simulink model "FuzzyHYPFWMLI"  (R2025a)
settings: Solver=ode23t  StartTime=0.0  StopTime=1  FixedStep=1.0000000100000003E-5  MaxStep=1e-3  RelTol=1e-2  EnableMultiTasking=on
undefined symbols (not defined in the file): c1, c2, c3, c4, c5, c6, DiscIntNeverNeededParam, FC1, FC2, idq1, idq2, PV10k1, PV10k2, PV10k3, R, WM1
libraries: powerlib x93, powerlib_meascontrol x9, fuzblock x8, powerlib_extras x6, re_lib x3, electricdrivelib x2, slpidlib x1
(part 2 of 3)

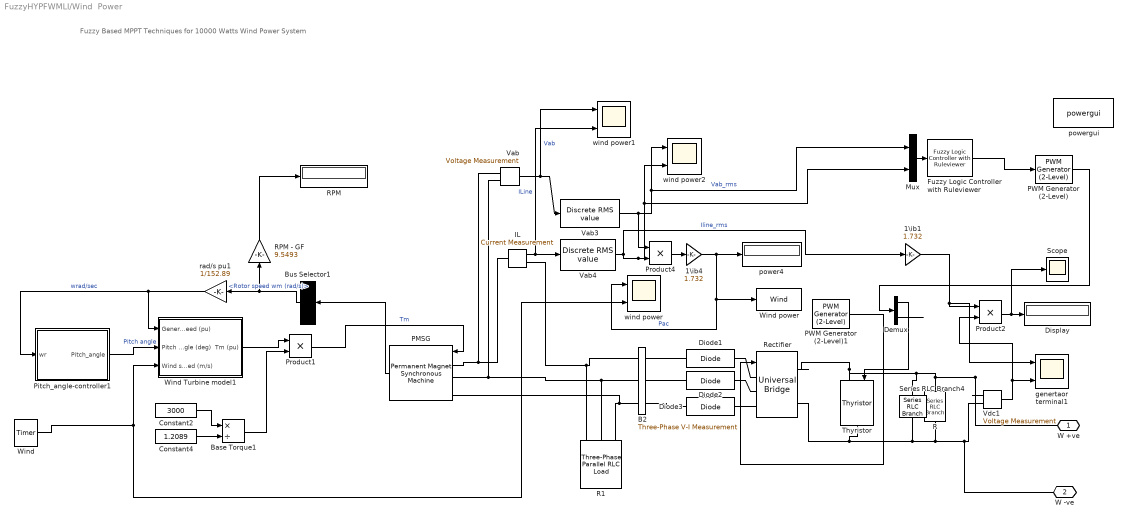
== system FuzzyHYPFWMLI/Wind  Power  ==
  note: Fuzzy Based MPPT Techniques for 10000 Watts Wind Power System
  1\ib1 : Gain  Gain=1.732  SaturateOnIntegerOverflow=on  OutDataTypeStr=Inherit: Same as input  ParamDataTypeStr=Inherit: Same as input
  1\ib4 : Gain  Gain=1.732  SaturateOnIntegerOverflow=on  OutDataTypeStr=Inherit: Same as input  ParamDataTypeStr=Inherit: Same as input
  "B2 " : powerlib/Measurements/Three-Phase V-I Measurement  VoltageMeasurement=no  SetLabelV=on  LabelV=Vabc_B2  Vpu=off  VpuLL=off  CurrentMeasurement=no  SetLabelI=on  LabelI=Iabc_B2  Ipu=off  Pbase=100e6  Vbase=500e3  OutputType=Magnitude  PhasorSimulation=off  PSBequivalent=0
  Base Torque1 : Product  Inputs=*/  RndMeth=Zero
  Bus Selector1 : BusSelector  OutputSignals=Rotor speed wm (rad/s)
  Constant2 : Constant  Value=3000
  Constant4 : Constant  Value=1.2089
  Demux : Demux  Outputs=2
  Diode1 : powerlib/Power Electronics/Diode  Ron=0.001  Lon=0  Vf=0.8  IC=0  UseSnubber=off  Rs=500  Cs=250e-9  Measurements=off
  Diode2 : powerlib/Power Electronics/Diode  Ron=0.001  Lon=0  Vf=0.8  IC=0  UseSnubber=off  Rs=500  Cs=250e-9  Measurements=off
  Diode3 : powerlib/Power Electronics/Diode  Ron=0.001  Lon=0  Vf=0.8  IC=0  UseSnubber=off  Rs=500  Cs=250e-9  Measurements=off
  Display : Display
  Fuzzy Logic Controller with Ruleviewer : fuzblock/Fuzzy Logic  Controller  with Ruleviewer  fismatrix=[WM1]  Ts=0.01
  IL : powerlib/Measurements/Current Measurement  PhasorSimulation=off  OutputType=Complex  PSBequivalent=0
  Mux : Mux  Inputs=2
  PMSG : powerlib/Machines/Permanent Magnet Synchronous Machine  NbPhases=3  FluxDistribution=Sinusoidal  RotorType=Round  MechanicalLoad=Torque Tm  PresetModel=No  ShowDetailedParameters=on  MeasurementBus=off  Resistance=0.0918  Inductance=8.5e-3  dqInductances=[0.0082 0.0082]  La=0.000975  MachineConstant=Flux linkage established by magnets (V.s)  Flux=0.1688  VoltageCst=122.4677  TorqueCst=1.0128  Flat=120  Mechanical=[0.003945 0.0004924 4 0]  PolePairs=4  InitialConditions=[0,0, 0,0]  InitialConditions5ph=[0 0 0 0 0 0]  TsPowergui=0  TsBlock=-1  RefAngle=90 degrees behind phase A axis (modified Park)
      settings: SourceProductName=Simscape Power Systems
  PWM Generator (2-Level) : powerlib_meascontrol/Pulse & Signal Generators/PWM Generator (2-Level)  ModulatorType=Single-phase half-bridge (2 pulses)  ModulatorMode=Unsynchronized  Fc=3000  Pc=90  nF=27  MinMax="[ -1  1 ]"  SamplingTechnique=Natural  ModulatingSignals=off  m=0.8  Freq=60  Phase=0  Ts=0  ShowCarrierOutport=off
      settings: SourceProductName=Simscape Power Systems
  PWM Generator (2-Level)1 : powerlib_meascontrol/Pulse & Signal Generators/PWM Generator (2-Level)  ModulatorType=Three-phase bridge (6 pulses)  ModulatorMode=Unsynchronized  Fc=27*60  Pc=90  nF=27  MinMax="[ -1  1 ]"  SamplingTechnique=Natural  ModulatingSignals=on  m=0.7  Freq=50  Phase=0  Ts=0  ShowCarrierOutport=off
      settings: SourceProductName=Simscape Power Systems
  Pitch_angle-controller1 : Subsystem
  Product1 : Product  RndMeth=Zero
  Product2 : Product  RndMeth=Zero
  Product4 : Product  RndMeth=Zero
  R : powerlib/Elements/Series RLC Branch  LConnTagsString=__new0  RConnTagsString=__new0  BranchType=R  Resistance=10e3  Inductance=1e-3  SetiL0=off  InitialCurrent=0  Capacitance=1e-6  Setx0=off  InitialVoltage=0  Measurements=None
  "R1 " : powerlib/Elements/Three-Phase Parallel RLC Load  LConnTagsString=A|B|C  Configuration=Y (grounded)  NominalVoltage=220  Vabc=[1e3 1e3 1e3]  Vabcp=[1e3 1e3 1e3]  NominalFrequency=50  UnbalancedPower=off  ActivePower=12000  InductivePower=0  CapacitivePower=0  Pabc=[9e3 9e3 9e3]  QLabc=[100 90 110]  QCabc=[100 90 110]  Pabcp=[10e3 9e3 11e3]  QLabcp=[100 90 110]  QCabcp=[100 90 110]  Measurements=None  LoadType=constant Z
  "RPM " : Display
  RPM - GF : Gain  Gain=9.5493  SaturateOnIntegerOverflow=on  OutDataTypeStr=Inherit: Same as input  ParamDataTypeStr=Inherit: Same as input
  Rectifier : powerlib/Power Electronics/Universal Bridge  Arms=3  SnubberResistance=100  SnubberCapacitance=0.1e-6  Device=IGBT / Diodes  Ron=1e-3  Lon=0  ForwardVoltages="[  100  100  ]"  ForwardVoltage=.8  GTOparameters=[ 10e-6 , 20e-6 ]  IGBTparameters=[ 1e-6 , 2e-6 ]  Measurements=Device currents  Measurements_2=None  converterType=Rectifier
  Scope : Scope
      settings: Title=Fuzzy Wind MPPT  ActiveDisplayYMinimum=-1251.33886  ActiveDisplayYMaximum=11262.04974  YLabel=Power ( W )
  Series RLC Branch4 : powerlib/Elements/Series RLC Branch  LConnTagsString=__new0  RConnTagsString=__new0  BranchType=C  Resistance=R  Inductance=1e-3  SetiL0=off  InitialCurrent=0  Capacitance=470e-5  Setx0=off  InitialVoltage=0  Measurements=Branch voltage and current
  Thyristor : powerlib/Power Electronics/Thyristor  Ron=0.001  Lon=0  Vf=220  IC=0  Rs=500  Cs=250e-9  Measurements=off
  Vab : powerlib/Measurements/Voltage Measurement  PhasorSimulation=off  OutputType=Complex  PSBequivalent=0
  Vab3 : powerlib_extras/Discrete Measurements/Discrete  RMS value  Freq=50  Mag_Init=0  Ts=20e-6
  Vab4 : powerlib_extras/Discrete Measurements/Discrete  RMS value  Freq=50  Mag_Init=0  Ts=20e-6
  Vdc1 : powerlib/Measurements/Voltage Measurement  Tag=PoWeRsYsTeMmEaSuReMeNt  PhasorSimulation=off  OutputType=Magnitude  PSBequivalent=0
  "Wind " : powerlib_extras/Control  Blocks/Timer  t=[0 0.05 0.1 0.15 0.2 ]  e=[5 7 11 12 12]
  Wind Turbine model1 : Subsystem  AncestorBlock=DRlib/Wind Generation/Wind Turbine  DialogController=POWERSYS.PowerSysDialog  mask(Wind Turbine){Pnom=10000, Pelec_base=10000/0.9, wind_base=12, P_wind_base=0.8, speed_nom=1, pitch_angle=0, DisplayTurbChar=off, c1_c6=[0.51763          116          0.4            5           21     0.006795], cp_nom=0.48, lambda_nom=8.1}
      mask prompts: Pnom "Nominal mechanical output power (W):"; Pelec_base "Base power of the electrical generator (VA):"; wind_base "Base wind speed (m/s):"; P_wind_base "Maximum power at base wind speed (pu of nominal mechanical power):"; speed_nom "Base rotational speed (p.u. of base generator speed):"; pitch_angle "Pitch angle beta to display wind-turbine power characteristics (beta >=0)  (deg):"; DisplayTurbChar "Display wind turbine power characteristics"
      mask help:
      | This block implements a variable pitch wind turbine model. The performance coefficient Cp of the turbine is the mechanical output power of the turbine divided by wind power and a function of wind speed, rotational speed, and pitch angle (beta). Cp reaches its maximum value at zero beta. Select the wind-turbine power characteristics display to plot the turbine characteristics at the specified pitch angle.
      |
      | The first input is the generator speed in per unit of the generator base speed. For a synchronous or asynchronous generator, the base speed is the synchronous speed. For a permanent-magnet generator, the base speed is defined as the speed producing nominal voltage at  no load. The second input is the blade pitch angle (beta) in degrees. The third input is the wind speed in m/s.
      |
      | The output is the torque applied to the generator shaft in per unit of the generator ratings.
      |
      | The turbine inertia must be added to the generator inertia.
      mask init:
      | %Wind turbine typical characteristic data
      | %c2=116;c3=0.4;c4=5;c5=21;
      | %Computation of c1 and c6 for lambda_nom et cpmax
      | %lambda_nom=8.1;
      | %cp_max=0.48;
      | %cp_nom=cp_max;
      | 
      | %lambda_i_nom=1/(1/lambda_nom-0.035);
      | %k_nom=-(c2*c5/lambda_i_nom-c4*c5-c2)*exp(-c5/lambda_i_nom)/lambda_nom^2;
      | %c1=cp_max/((c2/lambda_i_nom-c4)*exp(-c5/lambda_i_nom)+k_nom*lambda_nom);
      | %c6=k_nom*c1;
      | power_initmask();
      mask Help: web(psbhelp);
      mask Callback Pnom:
      | ParVisible={'on','on','on','on','on','on','on','off','off','off',};
      | set_param(gcb,'MaskVisibilities',ParVisible);
      | c1_c6=str2num(get_param(gcb,'c1_c6'));
      | c1=c1_c6(1);c2=c1_c6(2);c3=c1_c6(3);c4=c1_c6(4);c5=c1_c6(5);c6=c1_c6(6);
      mask Callback DisplayTurbChar:
      | DisplayTurbChar=get_param(gcb,'DisplayTurbChar');
      | 
      | if strcmp(DisplayTurbChar,'on')
      |     fig_num=figure;
      | 	clf(fig_num);
      | 	[speed_nom,wind_base,P_wind_base,pitch_angle]=getSPSmaskvalues(gcb,{'speed_nom','wind_base','P_wind_base','pitch_angle'});
      | 	[c1_c6,lambda_nom,cp_nom]=getSPSmaskvalues(gcb,{'c1_c6','lambda_nom','cp_nom'});
      | 	c1=c1_c6(1);c2=c1_c6(2);c3=c1_c6(3);c4=c1_c6(4);c5=c1_c6(5);c6=c1_c6(6);
      | 
      | 	%Wind turbine typical characteristic data
      |     %c2=116;c3=0.4;c4=5;c5=21;
      |     %Computation of c1 and c6 for lambda_nom et cpmax
      |     %lambda_nom=8.1;
      |     %cp_max=0.48;
      |     %cp_nom=cp_max;
      | 
      |     %lambda_i_nom=1/(1/lambda_nom-0.035);
      |     %k_nom=-(c2*c5/lambda_i_nom-c4*c5-c2)*exp(-c5/lambda_i_nom)/lambda_nom^2;
      |     %c1=cp_max/((c2/lambda_i_nom-c4)*exp(-c5/lambda_i_nom)+k_nom*lambda_nom);
      |     %c6=k_nom*c1;
      | 
      | 	wr_elec_pu=1e-3:0.01:1.5;;
      |     wr_mec_pu=wr_elec_pu/speed_nom;
      |     wind_max=ceil((1.2/P_wind_base)^(1/3)*wind_base);
      |     wind_min=round(((0.1)/P_wind_base)^(1/3)*wind_base);
      |     wind1=wind_min:(wind_base-wind_min)/5:wind_base;
      |     wind2=wind_base+(wind_base-wind_min)/5:(wind_base-wind_min)/5:wind_max;
      |     wind_pu=[wind1 wind2]/wind_base;
      | 
      |     for k=1:length(wind_pu)
      |         for i=1:length(wr_mec_pu);
      |             lambda_pu=wr_mec_pu(i)/wind_pu(k);
      |             lambda=lambda_pu*lambda_nom;
      |             lambda_i=1/(1/(lambda+0.08*pitch_angle)-0.035/(pitch_angle^3+1));
      |             cp=c1*(c2/lambda_i-c3*pitch_angle-c4)*exp(-c5/lambda_i)+c6*lambda;
      |             cp_pu=cp/cp_nom;
      |             Pwind_pu(k,i)=wind_pu(k)^3*cp_pu*P_wind_base;
      |         end
      |     end
      |     for k=1:length(wind_pu)
      |         plot(wr_elec_pu,Pwind_pu(k,:))
      |         hold on
      |     end
      | 
      |     plot([speed_nom,speed_nom,0],[0,P_wind_base,P_wind_base],'r--')
      |     text(speed_nom+0.01,0+0.05,sprintf('%0.4g pu',speed_nom))
      |     text(0.01,P_wind_base+0.05,sprintf('Max. power at base wind speed (%0.4g m/s) and beta = 0 deg',wind_base))
      |     for i=1:length(wind_pu),
      |         p_max(i)=max(Pwind_pu(i,:));
      |         speed(i)=wr_elec_pu(find(Pwind_pu(i,:)==p_max(i)));
      |         text(speed(i),p_max(i),sprintf('%0.4g m/s',wind_pu(i)*wind_base))
      |     end
      |     plot([0 max(wr_elec_pu)],[0 0],'--')
      | 
      |     xlabel('Turbine speed (pu of nominal generator speed)')
      |     ylabel('Turbine output power (pu of nominal mechanical power)')
      |     title(sprintf('Turbine Power Characteristics (Pitch angle beta = %0.4g deg)',pitch_angle))
      |     axis([0 max(wr_elec_pu) min(Pwind_pu(1,:)) max(P_wind_base+0.1,max(wind_pu)^3*P_wind_base+0.1)])
      |     set_param(gcb,'DisplayTurbChar','off')
      | end
      mask Display: disp('');
  Wind power : ToWorkspace  VariableName=Wind  SaveFormat=Timeseries  SampleTime=-1
  genertaor terminal1 : Scope  NumInputPorts=2
      settings: SampleTime=100e-6  ActiveDisplayYMinimum=-6.25669  ActiveDisplayYMaximum=56.31021  DataLoggingVariableName=ScopeData2
  power4 : Display
      settings: SampleTime=1e-3
  powergui : powerlib/powergui  Priority=1  SimulationMode=Discrete  SampleTime=50e-6  frequency=60  Iterations=50  frequencyindice=0  Pbase=100e6  ErrMax=1e-4  UnitsV=kV  UnitsW=MW  buscounter=0  FunctionMessages=off  echomessages=off  EnableUseOfTLC=off  CurrentSourceSwitches=off  DisableSnubberDevices=off  DisableRonSwitches=off  DisableVfSwitches=off  DisplayEquations=off  SolverType=Tustin/Backward Euler (TBE)  Interpol=off  ExternalGateDelay=off  methode=off  Ts=100  x0status=blocks  SPID=off  SwTol=0  HookPort=off  RestoreLinks=warning  ResistiveCurrentMeasurement=off  Frange=[0:2:500]  Ylog=off  Xlog=on  ShowGrid=off  save=off  variable=ZData  structure=0  ZoomFFT=off  StartTime=0.0  cycles=1  DisplayStyle=1  fundamental=60  FreqAxis=off  MaxFrequency=1000  frequencyindicesteady=1  RmsSteady=1  display=off
  rad/s pu1 : Gain  Gain=1/152.89  SaturateOnIntegerOverflow=on  OutDataTypeStr=Inherit: Same as input  ParamDataTypeStr=Inherit: Same as input
  wind power : Scope  NumInputPorts=2
      settings: SampleTime=100e-6  Title=Power Wind  ActiveDisplayYMinimum=-1255.48273  ActiveDisplayYMaximum=11299.34461  YLabel=Power ( W )  DataLoggingVariableName=ScopeData3
  wind power1 : Scope  NumInputPorts=2
      settings: SampleTime=100e-6  ActiveDisplayYMinimum=-365.65456  ActiveDisplayYMaximum=365.65434  DataLoggingVariableName=ScopeData4
  wind power2 : Scope  NumInputPorts=2
      settings: SampleTime=100e-6  ActiveDisplayYMinimum=-25.23289  ActiveDisplayYMaximum=227.09602  YLabel=Voltage( V )  DataLoggingVariableName=ScopeData5
  W +ve : PMIOPort  Side=Right
  W -ve : PMIOPort  Port=2  Side=Right
  wires:
  Vdc1/1 -> genertaor terminal1/2, Product2/2
  Bus Selector1/1 -> RPM - GF/1, rad/s pu1/1  "<Rotor speed wm (rad/s)>"
  1\ib4/1 -> power4/1, Wind power/1, wind power/1  "Pac"
  IL/1 -> wind power1/2, Vab4/1  "ILine"
  Product2/1 -> Scope/1, Display/1
  Wind Turbine model1/1(Tm (pu)) -> Product1/1
  Vab4/1 -> 1\ib1/1, Mux/2, wind power2/2, Product4/2  "Iline_rms"
  Demux/1 -> Thyristor/1
  Mux/1 -> Fuzzy Logic Controller with Ruleviewer/1
  Vab/1 -> wind power1/1, Vab3/1  "Vab"
  Constant2/1 -> Base Torque1/1
  "Wind "/1 -> Wind Turbine model1/3(Wind speed (m/s)), wind power/2
  Pitch_angle-controller1/1(Pitch_angle) -> Wind Turbine model1/2(Pitch angle (deg))  "Pitch angle"
  rad/s pu1/1 -> Pitch_angle-controller1/1(wr), Wind Turbine model1/1(Generator speed (pu))  "wrad/sec"
  PWM Generator (2-Level)1/1 -> Rectifier/1
  Product1/1 -> PMSG/1  "Tm"
  Vab3/1 -> Product4/1, Mux/1, wind power2/1  "Vab_rms"
  1\ib1/1 -> genertaor terminal1/1, Product2/1
  RPM - GF/1 -> "RPM "/1
  Constant4/1 -> Base Torque1/2
  PMSG/1 -> Bus Selector1/1
  Product4/1 -> 1\ib4/1
  Fuzzy Logic Controller with Ruleviewer/1 -> PWM Generator (2-Level)/1
  Base Torque1/1 -> Product1/2
  PWM Generator (2-Level)/1 -> Demux/1
  Demux/2 -> ?
  connections:
  Vdc1/LConn2 -- R/RConn1 -- Series RLC Branch4/RConn1 -- Thyristor/RConn1 -- Rectifier/RConn2 -- W -ve/RConn1
  Diode1/LConn1 -- "B2 "/RConn1
  Vdc1/LConn1 -- Series RLC Branch4/LConn1 -- Thyristor/LConn1 -- Rectifier/RConn1 -- R/LConn1 -- W +ve/RConn1
  "B2 "/LConn2 -- "R1 "/LConn2 -- PMSG/LConn2 -- Vab/LConn2
  "B2 "/LConn1 -- "R1 "/LConn1 -- IL/RConn1
  Vab/LConn1 -- IL/LConn1 -- PMSG/LConn1
  Diode3/RConn1 -- Rectifier/LConn3
  PMSG/LConn3 -- "R1 "/LConn3 -- "B2 "/LConn3
  Diode2/RConn1 -- Rectifier/LConn2
  Diode2/LConn1 -- "B2 "/RConn2
  Diode1/RConn1 -- Rectifier/LConn1
  "B2 "/RConn3 -- Diode3/LConn1

== system FuzzyHYPFWMLI/Fuel Cell 1/100Vdc Boost DC//DC Converter (average value) ==
  CBus : powerlib/Elements/Series RLC Branch  LConnTagsString=__new0  RConnTagsString=__new0  BranchType=RC  Resistance=0.2  Inductance=1e-3  SetiL0=off  InitialCurrent=0  Capacitance=7500e-6  Setx0=on  InitialVoltage=100  Measurements=None
  Chopper : Subsystem  mask(SPSdrives Converter){SnubberResistance=10e3, SnubberCapacitance=inf, Ron=1e-3, ForwardVoltages=[1.3,1.3], IGBTParameters=[0,0], converterType=Inverter}
      mask prompts: SnubberResistance "Snubber resistance Rs (Ohms):"; SnubberCapacitance "Snubber capacitance Cs (F):"; Ron "Ron (Ohms):"; ForwardVoltages "Forward voltages [Device Vf(V), Diode Vd (V)]"; IGBTParameters "[Tf(s), Tt(s)]:"; converterType "Converter type:"
      mask help: This model implements an average-value buck converter."Duty Cycle" contains the duty cycle of the internal IGBT device.
      mask TypeOptions converterType: Rectifier | Inverter
      mask Display: plot(0,0,100,100,[39 39 23.8],[71 28 28],[44 56 49.6 56 52.8 56 61 61],[39.2 33.6 32.8 33.6 40.8 33.6 30 12.4],[44 44 44 61 61],[28 71 60 66.4 90],[75 67 83 75 67 83 75 75],[54 42 42 54 54 54 54 66],[61 75 75],[24 24 42],[75 75 61],[66,76,76])
  Constant : Constant  Value=100
  Current controller DISCRETE1 : Subsystem  mask(PI controller){Kp=0.0005, Ki=0.15, Ts=1e-3}
      mask prompts: Kp "Proportional gain (Kp)"; Ki "Integral gain (Ki)"; Ts "Sample time (s) :"
      mask help: Proportional-Integral Speed Controller
      mask Display: plot(0,0,100,100,[35,35,65],[70,30,30],[35,65],[45,60])
  Duty Cycles : Subsystem
  L : powerlib/Elements/Series RLC Branch  LConnTagsString=__new0  RConnTagsString=__new0  BranchType=L  Resistance=0.3  Inductance=500e-6  SetiL0=off  InitialCurrent=0  Capacitance=100e-6  Setx0=off  InitialVoltage=0  Measurements=None
  Transfer Fcn : TransferFcn  Denominator=[0.001 1]
  Voltage Measurement : powerlib/Measurements/Voltage Measurement  PhasorSimulation=off  OutputType=Complex  PSBequivalent=0
  + : PMIOPort  Tag=PMCPort  Side=Right
  - : PMIOPort  Tag=PMCPort  Port=2  Side=Right
  + FC : PMIOPort  Tag=PMCPort  Port=3  Side=Left
  - FC : PMIOPort  Tag=PMCPort  Port=4  Side=Left
  wires:
  Current controller DISCRETE1/1(Ec) -> Duty Cycles/1(Ec)
  Transfer Fcn/1 -> Current controller DISCRETE1/1(UBus)
  Duty Cycles/1(dc) -> Chopper/1(Duty Cycle)
  Voltage Measurement/1 -> Transfer Fcn/1
  Constant/1 -> Current controller DISCRETE1/2(Uref)
  connections:
  + FC/RConn1 -- L/RConn1
  Chopper/RConn1 -- L/LConn1
  CBus/LConn1 -- Chopper/LConn1 -- +/RConn1 -- Voltage Measurement/LConn1
  Chopper/LConn2 -- CBus/RConn1 -- -/RConn1 -- Voltage Measurement/LConn2 -- - FC/RConn1

== system FuzzyHYPFWMLI/Fuel Cell 2/100Vdc Boost DC//DC Converter (average value) ==
  CBus : powerlib/Elements/Series RLC Branch  LConnTagsString=__new0  RConnTagsString=__new0  BranchType=RC  Resistance=0.2  Inductance=1e-3  SetiL0=off  InitialCurrent=0  Capacitance=7500e-6  Setx0=on  InitialVoltage=100  Measurements=None
  Chopper : Subsystem  mask(SPSdrives Converter){SnubberResistance=10e3, SnubberCapacitance=inf, Ron=1e-3, ForwardVoltages=[1.3,1.3], IGBTParameters=[0,0], converterType=Inverter}
      mask prompts: SnubberResistance "Snubber resistance Rs (Ohms):"; SnubberCapacitance "Snubber capacitance Cs (F):"; Ron "Ron (Ohms):"; ForwardVoltages "Forward voltages [Device Vf(V), Diode Vd (V)]"; IGBTParameters "[Tf(s), Tt(s)]:"; converterType "Converter type:"
      mask help: This model implements an average-value buck converter."Duty Cycle" contains the duty cycle of the internal IGBT device.
      mask TypeOptions converterType: Rectifier | Inverter
      mask Display: plot(0,0,100,100,[39 39 23.8],[71 28 28],[44 56 49.6 56 52.8 56 61 61],[39.2 33.6 32.8 33.6 40.8 33.6 30 12.4],[44 44 44 61 61],[28 71 60 66.4 90],[75 67 83 75 67 83 75 75],[54 42 42 54 54 54 54 66],[61 75 75],[24 24 42],[75 75 61],[66,76,76])
  Constant : Constant  Value=100
  Current controller DISCRETE1 : Subsystem  mask(PI controller){Kp=0.0005, Ki=0.15, Ts=1e-3}
      mask prompts: Kp "Proportional gain (Kp)"; Ki "Integral gain (Ki)"; Ts "Sample time (s) :"
      mask help: Proportional-Integral Speed Controller
      mask Display: plot(0,0,100,100,[35,35,65],[70,30,30],[35,65],[45,60])
  Duty Cycles : Subsystem
  L : powerlib/Elements/Series RLC Branch  LConnTagsString=__new0  RConnTagsString=__new0  BranchType=L  Resistance=0.3  Inductance=500e-6  SetiL0=off  InitialCurrent=0  Capacitance=100e-6  Setx0=off  InitialVoltage=0  Measurements=None
  Transfer Fcn : TransferFcn  Denominator=[0.001 1]
  Voltage Measurement : powerlib/Measurements/Voltage Measurement  PhasorSimulation=off  OutputType=Complex  PSBequivalent=0
  + : PMIOPort  Tag=PMCPort  Side=Right
  - : PMIOPort  Tag=PMCPort  Port=2  Side=Right
  + FC : PMIOPort  Tag=PMCPort  Port=3  Side=Left
  - FC : PMIOPort  Tag=PMCPort  Port=4  Side=Left
  wires:
  Constant/1 -> Current controller DISCRETE1/2(Uref)
  Voltage Measurement/1 -> Transfer Fcn/1
  Duty Cycles/1(dc) -> Chopper/1(Duty Cycle)
  Transfer Fcn/1 -> Current controller DISCRETE1/1(UBus)
  Current controller DISCRETE1/1(Ec) -> Duty Cycles/1(Ec)
  connections:
  - FC/RConn1 -- Voltage Measurement/LConn2 -- -/RConn1 -- CBus/RConn1 -- Chopper/LConn2
  Voltage Measurement/LConn1 -- +/RConn1 -- Chopper/LConn1 -- CBus/LConn1
  Chopper/RConn1 -- L/LConn1
  + FC/RConn1 -- L/RConn1

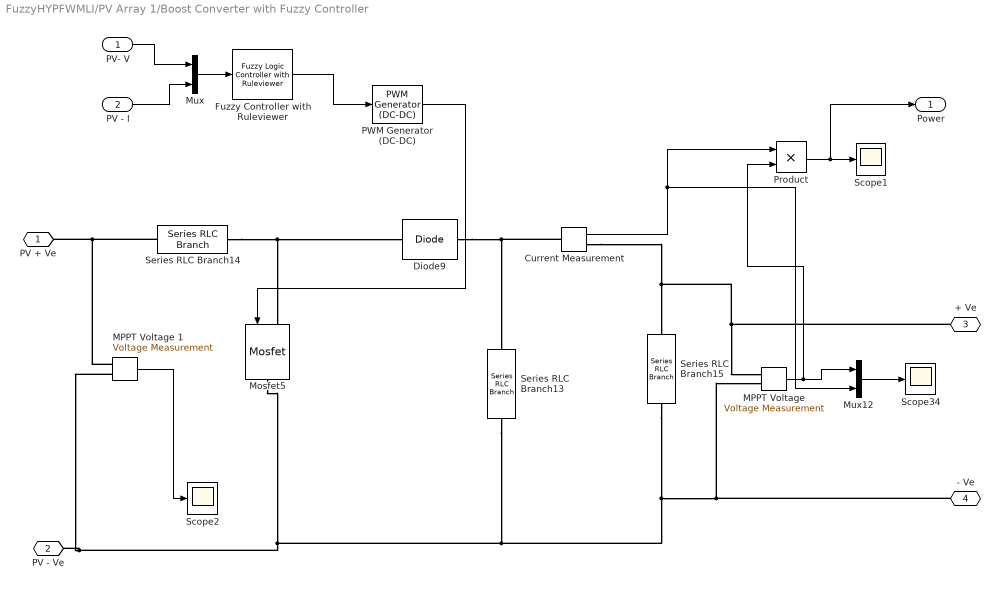
== system FuzzyHYPFWMLI/PV Array 1/Boost Converter with Fuzzy Controller ==
  " PV- V" : Inport
  PV - I : Inport  Port=2
  Current Measurement : powerlib/Measurements/Current Measurement  PhasorSimulation=off  OutputType=Complex  PSBequivalent=0
  Diode9 : powerlib/Power Electronics/Diode  Ron=0.001  Lon=0  Vf=0.8  IC=0  UseSnubber=off  Rs=500  Cs=250e-9  Measurements=off
  Fuzzy Controller with Ruleviewer : fuzblock/Fuzzy Logic  Controller  with Ruleviewer  fismatrix=[PV10k1]  Ts=0.01
  "MPPT Voltage " : powerlib/Measurements/Voltage Measurement  PhasorSimulation=off  OutputType=Complex  PSBequivalent=0
  MPPT Voltage 1 : powerlib/Measurements/Voltage Measurement  PhasorSimulation=off  OutputType=Complex  PSBequivalent=0
  Mosfet5 : powerlib/Power Electronics/Mosfet  Ron=0.1  Lon=0  Rd=0.01  Vfd=0  IC=0  Rs=1e5  Cs=inf  Measurements=off
  Mux : Mux  Inputs=2
  Mux12 : Mux  Inputs=2
  PWM Generator (DC-DC) : powerlib_meascontrol/Pulse & Signal Generators/PWM Generator (DC-DC)  Fsw=5000  Ts=0
  Product : Product
  Scope1 : Scope
      settings: Title=FUZZY BASED MPPT OF PV VOLTAGE AND CURRENT  ActiveDisplayYMinimum=-2375.71395  ActiveDisplayYMaximum=21381.47775  YLabel=Power ( W )  DataLoggingMaxPoints=50000000
  Scope2 : Scope
      settings: ActiveDisplayYMinimum=18.82  ActiveDisplayYMaximum=18.95  DataLoggingMaxPoints=50000000  DataLoggingVariableName=ScopeData6
  Scope34 : Scope
      settings: Title=FUZZY BASED MPPT OF PV VOLTAGE AND CURRENT  ActiveDisplayYMinimum=-23.8958  ActiveDisplayYMaximum=215.06216  YLabel=Voltage - Current  DataLoggingMaxPoints=50000000
  Series RLC Branch13 : powerlib/Elements/Series RLC Branch  LConnTagsString=__new0  RConnTagsString=__new0  BranchType=C  Resistance=1  Inductance=1e-3  SetiL0=off  InitialCurrent=0  Capacitance=550e-6  Setx0=off  InitialVoltage=0  Measurements=None
  Series RLC Branch14 : powerlib/Elements/Series RLC Branch  LConnTagsString=__new0  RConnTagsString=__new0  BranchType=L  Resistance=1  Inductance=0.05e-2  SetiL0=off  InitialCurrent=0  Capacitance=1e-6  Setx0=off  InitialVoltage=0  Measurements=None
  Series RLC Branch15 : powerlib/Elements/Series RLC Branch  LConnTagsString=__new0  RConnTagsString=__new0  BranchType=R  Resistance=13  Inductance=1e-3  SetiL0=off  InitialCurrent=0  Capacitance=1e-6  Setx0=off  InitialVoltage=0  Measurements=None
  PV + Ve : PMIOPort  Side=Left
  PV - Ve : PMIOPort  Port=2  Side=Left
  + Ve : PMIOPort  Port=3  Side=Right
  - Ve : PMIOPort  Port=4  Side=Right
  Power : Outport  VectorParamsAs1DForOutWhenUnconnected=off
  wires:
  MPPT Voltage 1/1 -> Scope2/1
  Mux12/1 -> Scope34/1
  "MPPT Voltage "/1 -> Product/2, Mux12/1
  " PV- V"/1 -> Mux/1
  Fuzzy Controller with Ruleviewer/1 -> PWM Generator (DC-DC)/1
  PWM Generator (DC-DC)/1 -> Mosfet5/1
  PV - I/1 -> Mux/2
  Product/1 -> Power/1, Scope1/1
  Mux/1 -> Fuzzy Controller with Ruleviewer/1
  Current Measurement/1 -> Mux12/2, Product/1
  connections:
  MPPT Voltage 1/LConn1 -- Series RLC Branch14/LConn1 -- PV + Ve/RConn1
  MPPT Voltage 1/LConn2 -- PV - Ve/RConn1 -- Series RLC Branch13/RConn1 -- - Ve/RConn1 -- "MPPT Voltage "/LConn2 -- Series RLC Branch15/RConn1 -- Mosfet5/RConn1
  Diode9/RConn1 -- Series RLC Branch13/LConn1 -- Current Measurement/LConn1
  Series RLC Branch14/RConn1 -- Diode9/LConn1 -- Mosfet5/LConn1
  + Ve/RConn1 -- "MPPT Voltage "/LConn1 -- Series RLC Branch15/LConn1 -- Current Measurement/RConn1

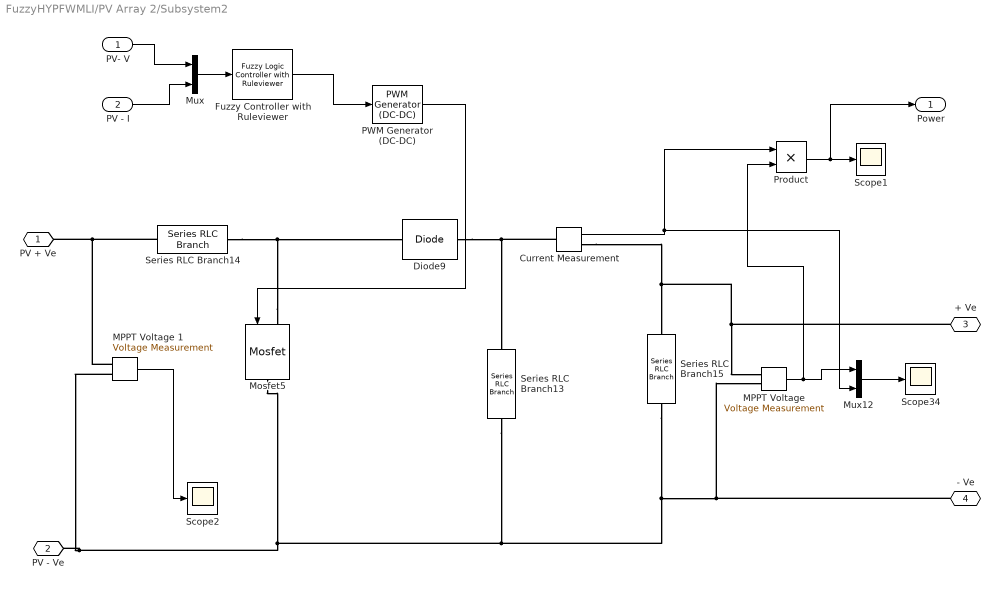
== system FuzzyHYPFWMLI/PV Array 2/Subsystem2 ==
  " PV- V" : Inport
  PV - I : Inport  Port=2
  Current Measurement : powerlib/Measurements/Current Measurement  PhasorSimulation=off  OutputType=Complex  PSBequivalent=0
  Diode9 : powerlib/Power Electronics/Diode  Ron=0.001  Lon=0  Vf=0.8  IC=0  UseSnubber=off  Rs=500  Cs=250e-9  Measurements=off
  Fuzzy Controller with Ruleviewer : fuzblock/Fuzzy Logic  Controller  with Ruleviewer  fismatrix=[PV10k2]  Ts=0.01
  "MPPT Voltage " : powerlib/Measurements/Voltage Measurement  PhasorSimulation=off  OutputType=Complex  PSBequivalent=0
  MPPT Voltage 1 : powerlib/Measurements/Voltage Measurement  PhasorSimulation=off  OutputType=Complex  PSBequivalent=0
  Mosfet5 : powerlib/Power Electronics/Mosfet  Ron=0.1  Lon=0  Rd=0.01  Vfd=0  IC=0  Rs=1e5  Cs=inf  Measurements=off
  Mux : Mux  Inputs=2
  Mux12 : Mux  Inputs=2
  PWM Generator (DC-DC) : powerlib_meascontrol/Pulse & Signal Generators/PWM Generator (DC-DC)  Fsw=5000  Ts=0
  Product : Product
  Scope1 : Scope
      settings: Title=FUZZY BASED MPPT OF PV VOLTAGE AND CURRENT  ActiveDisplayYMinimum=-2375.71395  ActiveDisplayYMaximum=21381.47775  YLabel=Power ( W )  DataLoggingMaxPoints=50000000
  Scope2 : Scope
      settings: ActiveDisplayYMinimum=18.82  ActiveDisplayYMaximum=18.95  DataLoggingMaxPoints=50000000  DataLoggingVariableName=ScopeData6
  Scope34 : Scope
      settings: Title=FUZZY BASED MPPT OF PV VOLTAGE AND CURRENT  ActiveDisplayYMinimum=-23.8958  ActiveDisplayYMaximum=215.06216  YLabel=Voltage - Current  DataLoggingMaxPoints=50000000
  Series RLC Branch13 : powerlib/Elements/Series RLC Branch  LConnTagsString=__new0  RConnTagsString=__new0  BranchType=C  Resistance=1  Inductance=1e-3  SetiL0=off  InitialCurrent=0  Capacitance=550e-6  Setx0=off  InitialVoltage=0  Measurements=None
  Series RLC Branch14 : powerlib/Elements/Series RLC Branch  LConnTagsString=__new0  RConnTagsString=__new0  BranchType=L  Resistance=1  Inductance=0.05e-2  SetiL0=off  InitialCurrent=0  Capacitance=1e-6  Setx0=off  InitialVoltage=0  Measurements=None
  Series RLC Branch15 : powerlib/Elements/Series RLC Branch  LConnTagsString=__new0  RConnTagsString=__new0  BranchType=R  Resistance=13  Inductance=1e-3  SetiL0=off  InitialCurrent=0  Capacitance=1e-6  Setx0=off  InitialVoltage=0  Measurements=None
  PV + Ve : PMIOPort  Side=Left
  PV - Ve : PMIOPort  Port=2  Side=Left
  + Ve : PMIOPort  Port=3  Side=Right
  - Ve : PMIOPort  Port=4  Side=Right
  Power : Outport  VectorParamsAs1DForOutWhenUnconnected=off
  wires:
  Mux/1 -> Fuzzy Controller with Ruleviewer/1
  Product/1 -> Scope1/1, Power/1
  PV - I/1 -> Mux/2
  PWM Generator (DC-DC)/1 -> Mosfet5/1
  Fuzzy Controller with Ruleviewer/1 -> PWM Generator (DC-DC)/1
  " PV- V"/1 -> Mux/1
  "MPPT Voltage "/1 -> Mux12/1, Product/2
  Mux12/1 -> Scope34/1
  MPPT Voltage 1/1 -> Scope2/1
  Current Measurement/1 -> Mux12/2, Product/1
  connections:
  Mosfet5/LConn1 -- Diode9/LConn1 -- Series RLC Branch14/RConn1
  Diode9/RConn1 -- Current Measurement/LConn1 -- Series RLC Branch13/LConn1
  Mosfet5/RConn1 -- Series RLC Branch15/RConn1 -- "MPPT Voltage "/LConn2 -- - Ve/RConn1 -- Series RLC Branch13/RConn1 -- PV - Ve/RConn1 -- MPPT Voltage 1/LConn2
  PV + Ve/RConn1 -- Series RLC Branch14/LConn1 -- MPPT Voltage 1/LConn1
  "MPPT Voltage "/LConn1 -- + Ve/RConn1 -- Current Measurement/RConn1 -- Series RLC Branch15/LConn1

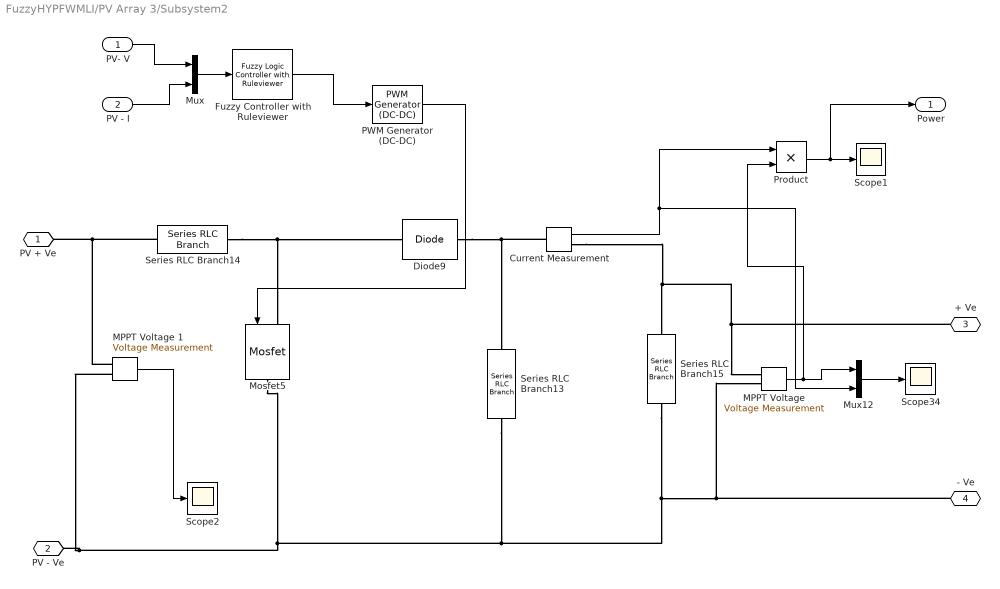
== system FuzzyHYPFWMLI/PV Array 3/Subsystem2 ==
  " PV- V" : Inport
  PV - I : Inport  Port=2
  Current Measurement : powerlib/Measurements/Current Measurement  PhasorSimulation=off  OutputType=Complex  PSBequivalent=0
  Diode9 : powerlib/Power Electronics/Diode  Ron=0.001  Lon=0  Vf=0.8  IC=0  UseSnubber=off  Rs=500  Cs=250e-9  Measurements=off
  Fuzzy Controller with Ruleviewer : fuzblock/Fuzzy Logic  Controller  with Ruleviewer  fismatrix=[PV10k3]  Ts=0.01
  "MPPT Voltage " : powerlib/Measurements/Voltage Measurement  PhasorSimulation=off  OutputType=Complex  PSBequivalent=0
  MPPT Voltage 1 : powerlib/Measurements/Voltage Measurement  PhasorSimulation=off  OutputType=Complex  PSBequivalent=0
  Mosfet5 : powerlib/Power Electronics/Mosfet  Ron=0.1  Lon=0  Rd=0.01  Vfd=0  IC=0  Rs=1e5  Cs=inf  Measurements=off
  Mux : Mux  Inputs=2
  Mux12 : Mux  Inputs=2
  PWM Generator (DC-DC) : powerlib_meascontrol/Pulse & Signal Generators/PWM Generator (DC-DC)  Fsw=5000  Ts=0
  Product : Product
  Scope1 : Scope
      settings: Title=FUZZY BASED MPPT OF PV VOLTAGE AND CURRENT  ActiveDisplayYMinimum=-2375.71395  ActiveDisplayYMaximum=21381.47775  YLabel=Power ( W )  DataLoggingMaxPoints=50000000
  Scope2 : Scope
      settings: ActiveDisplayYMinimum=18.82  ActiveDisplayYMaximum=18.95  DataLoggingMaxPoints=50000000  DataLoggingVariableName=ScopeData6
  Scope34 : Scope
      settings: Title=FUZZY BASED MPPT OF PV VOLTAGE AND CURRENT  ActiveDisplayYMinimum=-23.8958  ActiveDisplayYMaximum=215.06216  YLabel=Voltage - Current  DataLoggingMaxPoints=50000000
  Series RLC Branch13 : powerlib/Elements/Series RLC Branch  LConnTagsString=__new0  RConnTagsString=__new0  BranchType=C  Resistance=1  Inductance=1e-3  SetiL0=off  InitialCurrent=0  Capacitance=550e-6  Setx0=off  InitialVoltage=0  Measurements=None
  Series RLC Branch14 : powerlib/Elements/Series RLC Branch  LConnTagsString=__new0  RConnTagsString=__new0  BranchType=L  Resistance=1  Inductance=0.05e-2  SetiL0=off  InitialCurrent=0  Capacitance=1e-6  Setx0=off  InitialVoltage=0  Measurements=None
  Series RLC Branch15 : powerlib/Elements/Series RLC Branch  LConnTagsString=__new0  RConnTagsString=__new0  BranchType=R  Resistance=13  Inductance=1e-3  SetiL0=off  InitialCurrent=0  Capacitance=1e-6  Setx0=off  InitialVoltage=0  Measurements=None
  PV + Ve : PMIOPort  Side=Left
  PV - Ve : PMIOPort  Port=2  Side=Left
  + Ve : PMIOPort  Port=3  Side=Right
  - Ve : PMIOPort  Port=4  Side=Right
  Power : Outport  VectorParamsAs1DForOutWhenUnconnected=off
  wires:
  MPPT Voltage 1/1 -> Scope2/1
  Mux12/1 -> Scope34/1
  "MPPT Voltage "/1 -> Product/2, Mux12/1
  " PV- V"/1 -> Mux/1
  Fuzzy Controller with Ruleviewer/1 -> PWM Generator (DC-DC)/1
  PWM Generator (DC-DC)/1 -> Mosfet5/1
  PV - I/1 -> Mux/2
  Product/1 -> Power/1, Scope1/1
  Mux/1 -> Fuzzy Controller with Ruleviewer/1
  Current Measurement/1 -> Mux12/2, Product/1
  connections:
  MPPT Voltage 1/LConn1 -- Series RLC Branch14/LConn1 -- PV + Ve/RConn1
  MPPT Voltage 1/LConn2 -- PV - Ve/RConn1 -- Series RLC Branch13/RConn1 -- - Ve/RConn1 -- "MPPT Voltage "/LConn2 -- Series RLC Branch15/RConn1 -- Mosfet5/RConn1
  + Ve/RConn1 -- Current Measurement/RConn1 -- Series RLC Branch15/LConn1 -- "MPPT Voltage "/LConn1
  Series RLC Branch14/RConn1 -- Diode9/LConn1 -- Mosfet5/LConn1
  Diode9/RConn1 -- Current Measurement/LConn1 -- Series RLC Branch13/LConn1

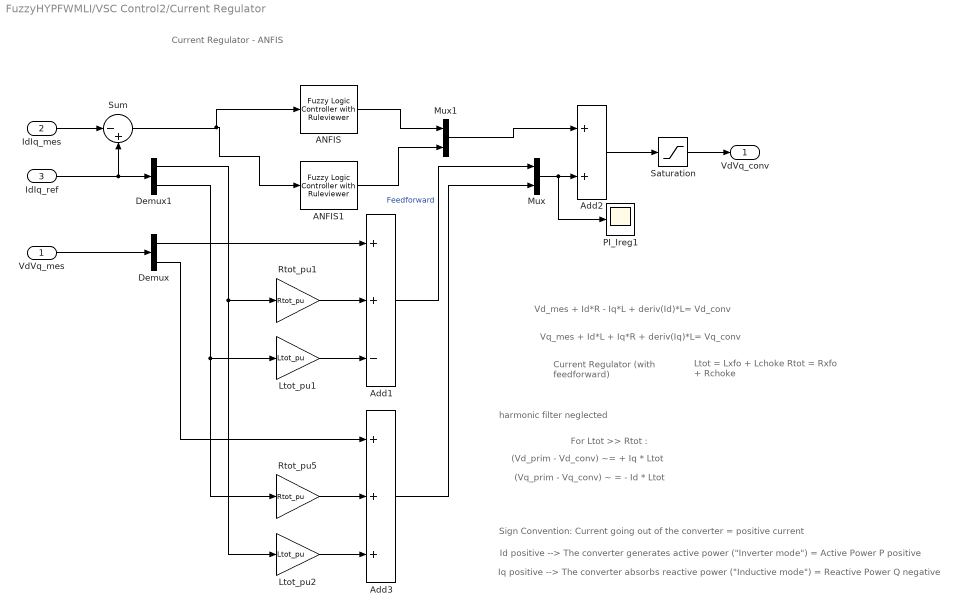
== system FuzzyHYPFWMLI/VSC Control2/Current Regulator ==
  note: Current Regulator - ANFIS
  note: harmonic filter neglected
  note: Vd_mes + Id*R - Iq*L + deriv(Id)*L= Vd_conv
  note: Vq_mes + Id*L + Iq*R + deriv(Iq)*L= Vq_conv
  note: Current Regulator
      | (with feedforward)
  note: Sign Convention: Current going out of the converter = positive current
  note: Iq positive --> The converter absorbs reactive power ("Inductive mode") = Reactive Power Q negative
  note: Id positive --> The converter generates active power ("Inverter mode") = Active Power P positive
  note: Ltot = Lxfo + Lchoke
      | Rtot = Rxfo + Rchoke
  note: (Vd_prim - Vd_conv) ~= + Iq * Ltot
  note: (Vq_prim - Vq_conv) ~ = - Id * Ltot
  note: For Ltot >> Rtot :
  VdVq_mes : Inport  PortDimensions=2
  IdIq_mes : Inport  Port=2  PortDimensions=2
  IdIq_ref : Inport  Port=3  PortDimensions=2
  ANFIS : fuzblock/Fuzzy Logic  Controller  with Ruleviewer  fismatrix=[idq1]  Ts=0.01
  ANFIS1 : fuzblock/Fuzzy Logic  Controller  with Ruleviewer  fismatrix=[idq2]  Ts=0.01
  Add1 : Sum  Inputs=++-
  Add2 : Sum
  Add3 : Sum  Inputs=+++
  Demux : Demux  Outputs=2
  Demux1 : Demux  Outputs=2
  Ltot_pu1 : Gain  Gain=Ltot_pu  SaturateOnIntegerOverflow=on  OutDataTypeStr=Inherit: Same as input  ParamDataTypeStr=Inherit: Same as input
  Ltot_pu2 : Gain  Gain=Ltot_pu  SaturateOnIntegerOverflow=on  OutDataTypeStr=Inherit: Same as input  ParamDataTypeStr=Inherit: Same as input
  Mux : Mux  Inputs=2
  Mux1 : Mux  Inputs=2
  PI_Ireg1 : Scope
      settings: TimeSpan=1  ActiveDisplayYMinimum=-0.4  ActiveDisplayYMaximum=1.1
  Rtot_pu1 : Gain  Gain=Rtot_pu  SaturateOnIntegerOverflow=on  OutDataTypeStr=Inherit: Same as input  ParamDataTypeStr=Inherit: Same as input
  Rtot_pu5 : Gain  Gain=Rtot_pu  SaturateOnIntegerOverflow=on  OutDataTypeStr=Inherit: Same as input  ParamDataTypeStr=Inherit: Same as input
  Saturation : Saturate  UpperLimit=2  LowerLimit=-2
  Sum : Sum  Inputs=|-+
  VdVq_conv : Outport  VectorParamsAs1DForOutWhenUnconnected=off
  wires:
  Mux/1 -> PI_Ireg1/1, Add2/2
  IdIq_ref/1 -> Sum/2, Demux1/1
  IdIq_mes/1 -> Sum/1
  Add2/1 -> Saturation/1
  Saturation/1 -> VdVq_conv/1
  VdVq_mes/1 -> Demux/1
  Demux/1 -> Add1/1
  Rtot_pu1/1 -> Add1/2
  Demux1/1 -> Rtot_pu1/1, Ltot_pu2/1
  Ltot_pu1/1 -> Add1/3
  Demux1/2 -> Ltot_pu1/1, Rtot_pu5/1
  Rtot_pu5/1 -> Add3/2
  Ltot_pu2/1 -> Add3/3
  Add1/1 -> Mux/1  "Feedforward"
  Demux/2 -> Add3/1
  Add3/1 -> Mux/2
  Sum/1 -> ANFIS1/1, ANFIS/1
  ANFIS/1 -> Mux1/1
  Mux1/1 -> Add2/1
  ANFIS1/1 -> Mux1/2

== system FuzzyHYPFWMLI/VSC Control2/PLL & Measurements ==
  note: Phase Lock Loop
  Vabc_prim : Inport
  Iabc_prim : Inport  Port=2
  PLL (3ph) : powerlib_meascontrol/PLL/PLL (3ph)  Fmin=45  Par_Init="[-0.57  Fnom]"  ParK=[180, 3200, 1]  TcD=1e-4  MaxRateChangeFreq=12  FilterCutOffFreq=25  Ts=Ts  AGC=on
  Selector1 : Selector  InputPortWidth=3  IndexOptions=Index vector (dialog)  Indices=[1 2]  OutputSizes=1
  Selector2 : Selector  InputPortWidth=3  IndexOptions=Index vector (dialog)  Indices=[1 2]  OutputSizes=1
  Terminator : Terminator
  V->pu : Gain  Gain=1/(Vnom_prim*sqrt(2)/sqrt(3))  SaturateOnIntegerOverflow=on  OutDataTypeStr=Inherit: Same as input  ParamDataTypeStr=Inherit: Same as input
  V->pu1 : Gain  Gain=Vnom_prim*sqrt(3)/Pnom/sqrt(2)  SaturateOnIntegerOverflow=on  OutDataTypeStr=Inherit: Same as input  ParamDataTypeStr=Inherit: Same as input
  abc to dq0 : powerlib_meascontrol/Transformations/abc to dq0  Alignment=90 degrees behind phase A axis
  abc to dq1 : powerlib_meascontrol/Transformations/abc to dq0  Alignment=90 degrees behind phase A axis
  wt : Outport  VectorParamsAs1DForOutWhenUnconnected=off
  VdVq_prim : Outport  Port=2  VectorParamsAs1DForOutWhenUnconnected=off
  IdIq_prim : Outport  Port=3  VectorParamsAs1DForOutWhenUnconnected=off
  wires:
  V->pu1/1 -> abc to dq1/1
  V->pu/1 -> PLL (3ph)/1, abc to dq0/1
  abc to dq1/1 -> Selector1/1
  Vabc_prim/1 -> V->pu/1
  Iabc_prim/1 -> V->pu1/1
  abc to dq0/1 -> Selector2/1
  Selector2/1 -> VdVq_prim/1
  Selector1/1 -> IdIq_prim/1
  PLL (3ph)/2 -> wt/1, abc to dq1/2, abc to dq0/2
  PLL (3ph)/1 -> Terminator/1

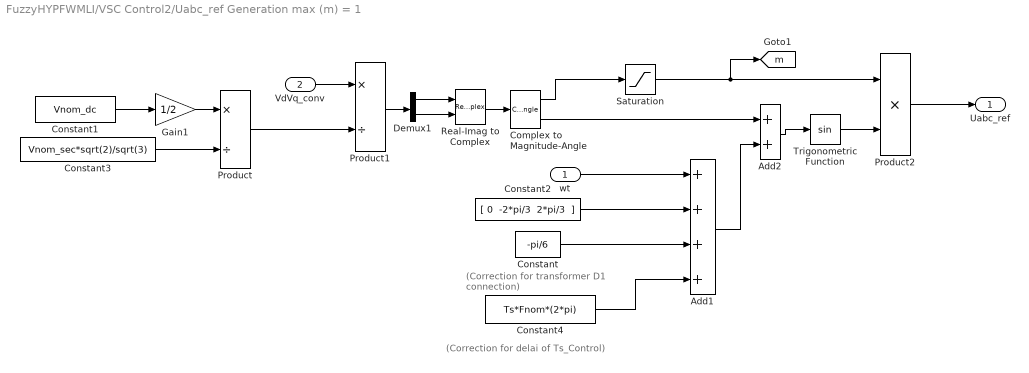
== system FuzzyHYPFWMLI/VSC Control2/Uabc_ref Generation max (m) = 1 ==
  note: (Correction for transformer
      |  D1 connection)
  note: (Correction for delai of Ts_Control)
  wt : Inport
  VdVq_conv : Inport  Port=2
  Add1 : Sum  Inputs=++++
  Add2 : Sum
  Complex to Magnitude-Angle : ComplexToMagnitudeAngle
  Constant : Constant  Value=-pi/6
  Constant1 : Constant  Value=Vnom_dc
  Constant2 : Constant  Value="[ 0  -2*pi/3  2*pi/3  ]"
  Constant3 : Constant  Value=Vnom_sec*sqrt(2)/sqrt(3)
  Constant4 : Constant  Value=Ts*Fnom*(2*pi)
  Demux1 : Demux  Outputs=2
  Gain1 : Gain  Gain=1/2
  Product : Product  Inputs=*/  RndMeth=Zero
  Product1 : Product  Inputs=*/  RndMeth=Zero
  Product2 : Product  Inputs=**  RndMeth=Zero
  Real-Imag to Complex : RealImagToComplex
  Saturation : Saturate  UpperLimit=1  LowerLimit=0
  Trigonometric Function : Trigonometry
  Uabc_ref : Outport  VectorParamsAs1DForOutWhenUnconnected=off
  tag scope: m=global
  wires:
  Complex to Magnitude-Angle/1 -> Saturation/1
  Constant1/1 -> Gain1/1
  VdVq_conv/1 -> Product1/1
  Product1/1 -> Demux1/1
  Gain1/1 -> Product/1
  Real-Imag to Complex/1 -> Complex to Magnitude-Angle/1
  Demux1/1 -> Real-Imag to Complex/1
  Demux1/2 -> Real-Imag to Complex/2
  Constant2/1 -> Add1/2
  Constant/1 -> Add1/3
  Constant3/1 -> Product/2
  Product/1 -> Product1/2
  Complex to Magnitude-Angle/2 -> Add2/1
  Add1/1 -> Add2/2
  Add2/1 -> Trigonometric Function/1
  Saturation/1 -> [m], Product2/1
  Trigonometric Function/1 -> Product2/2
  Product2/1 -> Uabc_ref/1
  wt/1 -> Add1/1
  Constant4/1 -> Add1/4

== system FuzzyHYPFWMLI/VSC Control2/VDC Regulator ==
  note: Voltage Regulator
  Vdc_mes : Inport  PortDimensions=1
  Vdc_ref : Inport  Port=2  PortDimensions=1
  PI : slpidlib/PID Controller  Controller=PI  Form=Parallel  TimeDomain=Discrete-time  UseExternalTs=off  SampleTime=Ts  IntegratorMethod=Trapezoidal  FilterMethod=Forward Euler  ControllerParametersSource=internal  P=Kp_VDCreg  I=Ki_VDCreg  UseKiTs=off  D=0  UseExternalDerivativeSource=off  N=100  UseFilter=on  TunerSelectOption=Transfer Function Based (PID Tuner App)  InitialConditionSource=internal  InitialConditionForIntegrator=0  InitialConditionForFilter=0  DifferentiatorICPrevScaledInput=0  ExternalReset=none  TrackingMode=off  Kt=1  LimitOutput=on  SatLimitsSource=internal  UpperSaturationLimit=1.5  LowerSaturationLimit=-1.5  LinearizeAsGain=off  AntiWindupMode=none  Kb=1  LimitIntegrator=off  UpperIntegratorSaturationLimit=inf  LowerIntegratorSaturationLimit=-inf  POutMin=[]  POutMax=[]  IOutMin=[]  IOutMax=[]  DOutMin=[]  DOutMax=[]  NOutMin=[]  NOutMax=[]  SumOutMin=[]  SumOutMax=[]  SaturationOutMin=[]  SaturationOutMax=[]  PParamMin=[]  PParamMax=[]  IParamMin=[]  IParamMax=[]  DParamMin=[]  DParamMax=[]  NParamMin=[]  NParamMax=[]  KbParamMin=[]  KbParamMax=[]  KtParamMin=[]  KtParamMax=[]  KbOutMin=[]  KbOutMax=[]  KtOutMin=[]  KtOutMax=[]  IntegratorOutMin=[]  IntegratorOutMax=[]  FilterOutMin=[]  FilterOutMax=[]  SumI1OutMin=[]  SumI1OutMax=[]  SumI2OutMin=[]  SumI2OutMax=[]  SumI3OutMin=[]  SumI3OutMax=[]  SumI4OutMin=[]  SumI4OutMax=[]  SumDOutMin=[]  SumDOutMax=[]  DifferentiatorOutMin=[]  DifferentiatorOutMax=[]  FilterDiffOutCoefMin=[]  FilterDiffOutCoefMax=[]  ReciprocalOutMin=[]  ReciprocalOutMax=[]  SumDenOutMin=[]  SumDenOutMax=[]  SumNumOutMin=[]  SumNumOutMax=[]  DivideOutMin=[]  DivideOutMax=[]  UdiffTsProdOutMin=[]  UdiffTsProdOutMax=[]  NTsProdOutMin=[]  NTsProdOutMax=[]  UintegralTsProdOutMin=[]  UintegralTsProdOutMax=[]  UngainTsProdOutMin=[]  UngainTsProdOutMax=[]  ClampingZeroOutDataTypeStr=Inherit: Inherit via back propagation  ClampingZeroOutMin=[]  ClampingZeroOutMax=[]  FilterDenConstantOutDataTypeStr=Inherit: Inherit via back propagation  FilterDenConstantOutMin=[]  FilterDenConstantOutMax=[]  PCopyOutDataTypeStr=Inherit: Inherit via back propagation  PCopyOutMin=[]  PCopyOutMax=[]  NCopyOutDataTypeStr=Inherit: Inherit via back propagation  NCopyOutMin=[]  NCopyOutMax=[]  IntegratorContinuousStateAttributes=''  IntegratorStateMustResolveToSignalObject=off  IntegratorRTWStateStorageClass=Auto  FilterContinuousStateAttributes=''  FilterStateMustResolveToSignalObject=off  FilterRTWStateStorageClass=Auto  ParallelPVariant=InternalParameters  IdealPVariant=Disabled  IVariant=InternalParameters  DVariant=Disabled  IntegratorVariant=Discrete  SatVariant=Enabled  AWVariant=Passthrough  PCopyVariant=Disabled  TRVariant=Disabled  FdbkBlocksVariant=Forward  IdealPFdbkVariant=Disabled  SatFdbkVariant=Disabled  DerivativeFilterVariant=Disabled  NVariant=Disabled  NCopyVariant=Disabled_SignalSpec  FilterICVariant=Disabled  IntegratorICVariant=InternalICs  ExternalResetVariant=Disabled  TRSumVariant=Passthrough  SumFdbkVariant=Disabled  SumVariant=Sum_PI  TsampFilterVariant=InternalTs  TsampNgainVariant=Passthrough  TsampIntegralVariant=Disabled_SignalSpec  ExternalSaturationOutDataTypeStr=Inherit: Same as second input  DerivativeSourceVariant=Disabled  PreIntVariant=InternalPreInt
  Rtot_pu3 : Gain  Gain=1/Vnom_dc  SaturateOnIntegerOverflow=on  OutDataTypeStr=Inherit: Same as input  ParamDataTypeStr=Inherit: Same as input
  Scope : Scope
      settings: ActiveDisplayYMinimum=-0.2  ActiveDisplayYMaximum=0.9  DataLoggingVariableName=ScopeData6  DataLoggingSaveFormat=Array
  Scope1 : Scope
      settings: ActiveDisplayYMinimum=-1.425  ActiveDisplayYMaximum=-1.575  DataLoggingVariableName=ScopeData7  DataLoggingSaveFormat=Array
  Scope2 : Scope  NumInputPorts=2
      settings: ActiveDisplayYMinimum=-1  ActiveDisplayYMaximum=-0.35  DataLoggingVariableName=ScopeData8  DataLoggingSaveFormat=Array
  Sum : Sum  Inputs=|+-
  Id_ref : Outport  SampleTime=Ts  InitialOutput=0  VectorParamsAs1DForOutWhenUnconnected=off
  tag scope: Id_ref=global, Vdc_ref=global
  wires:
  Sum/1 -> Rtot_pu3/1
  Vdc_mes/1 -> Sum/1
  Vdc_ref/1 -> Sum/2, [Vdc_ref]
  Rtot_pu3/1 -> Scope2/1, Scope/1, PI/1
  PI/1 -> Scope2/2, Scope1/1, [Id_ref], Id_ref/1

== system FuzzyHYPFWMLI/Wind  Power /Pitch_angle-controller1 ==
  wr : Inport
  0-pitch_max : Saturate  UpperLimit=45  LowerLimit=0
  Constant2 : Constant  Value=2
  "Rate Limiter   " : RateLimiter  RisingSlewLimit=2  FallingSlewLimit=-2
  Sum : Sum  Inputs=|+-  SaturateOnIntegerOverflow=on
  genertaor terminal6 : Scope  NumInputPorts=2
      settings: SampleTime=100e-6  ActiveDisplayYMinimum=-1  ActiveDisplayYMaximum=1  DataLoggingVariableName=ScopeData9
  pitch_gain : Gain  Gain=500  SaturateOnIntegerOverflow=on  OutDataTypeStr=Inherit: Same as input  ParamDataTypeStr=Inherit: Same as input
  Pitch_angle : Outport  VectorParamsAs1DForOutWhenUnconnected=off
  wires:
  wr/1 -> Sum/1
  0-pitch_max/1 -> genertaor terminal6/2, "Rate Limiter   "/1
  Constant2/1 -> Sum/2
  Sum/1 -> pitch_gain/1
  pitch_gain/1 -> 0-pitch_max/1
  "Rate Limiter   "/1 -> genertaor terminal6/1, Pitch_angle/1

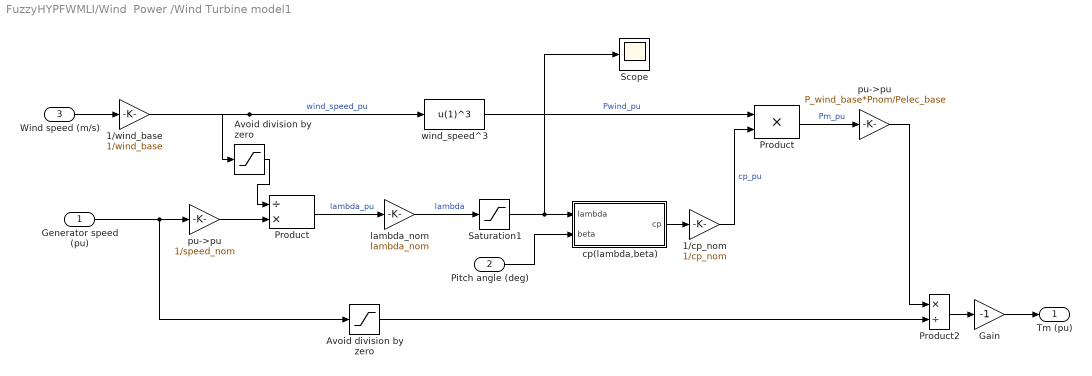
== system FuzzyHYPFWMLI/Wind  Power /Wind Turbine model1 ==
  Generator speed (pu) : Inport
  Pitch angle (deg) : Inport  Port=2
  Wind speed (m/s) : Inport  Port=3
  1/cp_nom : Gain  Gain=1/cp_nom  SaturateOnIntegerOverflow=on  OutDataTypeStr=Inherit: Same as input  ParamDataTypeStr=Inherit: Same as input
  1/wind_base : Gain  Gain=1/wind_base  SaturateOnIntegerOverflow=on  OutDataTypeStr=Inherit: Same as input  ParamDataTypeStr=Inherit: Same as input
  Avoid division by zero : Saturate  UpperLimit=1e6  LowerLimit=1e-6
  "Avoid division by zero " : Saturate  UpperLimit=1e6  LowerLimit=1e-6
  Gain : Gain  Gain=-1  SaturateOnIntegerOverflow=on  OutDataTypeStr=Inherit: Same as input  ParamDataTypeStr=Inherit: Same as input
  Product : Product  Inputs=/*  SaturateOnIntegerOverflow=on  OutDataTypeStr=Inherit: Same as first input
  "Product " : Product  SaturateOnIntegerOverflow=on  OutDataTypeStr=Inherit: Same as first input
  Product2 : Product  Inputs=*/  InputSameDT=on  SaturateOnIntegerOverflow=on  OutDataTypeStr=Inherit: Same as first input
  Saturation1 : Saturate  UpperLimit=inf  LowerLimit=1e-6
  Scope : Scope
      settings: DataLoggingVariableName=ScopeData10
  cp(lambda,beta) : Subsystem
  lambda_nom : Gain  Gain=lambda_nom  SaturateOnIntegerOverflow=on  OutDataTypeStr=Inherit: Same as input  ParamDataTypeStr=Inherit: Same as input
  pu->pu : Gain  Gain=P_wind_base*Pnom/Pelec_base  SaturateOnIntegerOverflow=on  OutDataTypeStr=Inherit: Same as input  ParamDataTypeStr=Inherit: Same as input
  "pu->pu " : Gain  Gain=1/speed_nom  SaturateOnIntegerOverflow=on  OutDataTypeStr=Inherit: Same as input  ParamDataTypeStr=Inherit: Same as input
  wind_speed^3 : Fcn  Expr=u(1)^3
  Tm (pu) : Outport  VectorParamsAs1DForOutWhenUnconnected=off
  wires:
  "pu->pu "/1 -> Product/2
  "Avoid division by zero "/1 -> Product/1
  1/wind_base/1 -> "Avoid division by zero "/1, wind_speed^3/1  "wind_speed_pu"
  Product/1 -> lambda_nom/1  "lambda_pu"
  Saturation1/1 -> Scope/1, cp(lambda,beta)/1(lambda)
  1/cp_nom/1 -> "Product "/2  "cp_pu"
  lambda_nom/1 -> Saturation1/1  "lambda"
  "Product "/1 -> pu->pu/1  "Pm_pu"
  Generator speed (pu)/1 -> "pu->pu "/1, Avoid division by zero/1
  Gain/1 -> Tm (pu)/1
  Wind speed (m/s)/1 -> 1/wind_base/1
  Avoid division by zero/1 -> Product2/2
  Product2/1 -> Gain/1
  wind_speed^3/1 -> "Product "/1  "Pwind_pu"
  cp(lambda,beta)/1(cp) -> 1/cp_nom/1
  pu->pu/1 -> Product2/1
  Pitch angle (deg)/1 -> cp(lambda,beta)/2(beta)

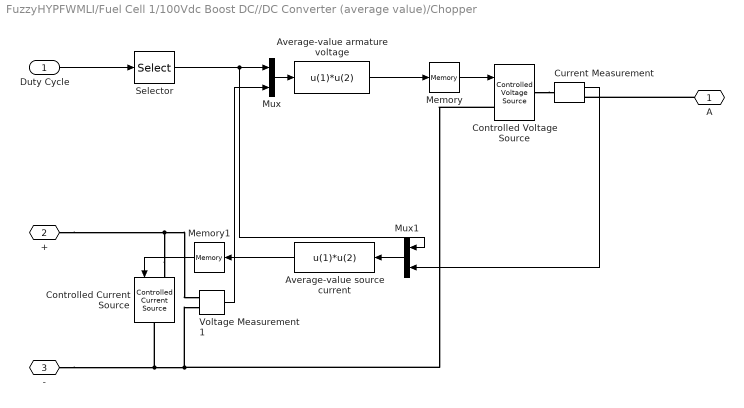
== system FuzzyHYPFWMLI/Fuel Cell 1/100Vdc Boost DC//DC Converter (average value)/Chopper ==
  Duty Cycle : Inport
  Average-value armature voltage : Fcn  Expr=u(1)*u(2)
  Average-value source current : Fcn  Expr=u(1)*u(2)
  Controlled Current Source : powerlib/Electrical Sources/Controlled Current Source  Initialize=on  Source_Type=AC  Amplitude=0  Phase=0  Frequency=0  Measurements=None
  Controlled Voltage Source : powerlib/Electrical Sources/Controlled Voltage Source  Initialize=on  Source_Type=AC  Amplitude=0  Phase=0  Frequency=0  Measurements=None
  Current Measurement : powerlib/Measurements/Current Measurement  Tag=PoWeRsYsTeMmEaSuReMeNt  PhasorSimulation=off  OutputType=Magnitude  PSBequivalent=0
  Memory : Memory
  Memory1 : Memory
  Mux : Mux  Inputs=2
  Mux1 : Mux  Inputs=2
  Selector : Selector  InputPortWidth=2  IndexOptions=Index vector (dialog)  Indices=[1]  OutputSizes=1
  Voltage Measurement1 : powerlib/Measurements/Voltage Measurement  Tag=PoWeRsYsTeMmEaSuReMeNt  PhasorSimulation=off  OutputType=Magnitude  PSBequivalent=0
  A : PMIOPort  Side=Right
  + : PMIOPort  Port=2  Side=Left
  - : PMIOPort  Port=3  Side=Left
  wires:
  Memory/1 -> Controlled Voltage Source/1
  Average-value armature voltage/1 -> Memory/1
  Mux/1 -> Average-value armature voltage/1
  Voltage Measurement1/1 -> Mux/2
  Duty Cycle/1 -> Selector/1
  Mux1/1 -> Average-value source current/1
  Current Measurement/1 -> Mux1/2
  Average-value source current/1 -> Memory1/1
  Memory1/1 -> Controlled Current Source/1
  Selector/1 -> Mux/1, Mux1/1
  connections:
  Voltage Measurement1/LConn2 -- Controlled Current Source/RConn1 -- -/RConn1 -- Controlled Voltage Source/LConn1
  Controlled Current Source/LConn1 -- Voltage Measurement1/LConn1 -- +/RConn1
  Controlled Voltage Source/RConn1 -- Current Measurement/LConn1
  A/RConn1 -- Current Measurement/RConn1

== system FuzzyHYPFWMLI/Fuel Cell 1/100Vdc Boost DC//DC Converter (average value)/Current controller DISCRETE1 ==
  UBus : Inport
  Uref : Inport  Port=2
  Ctrl sat. : Saturate  UpperLimit=0.95  LowerLimit=-0.95
  Discrete-Time Integrator : DiscreteIntegrator  IntegratorMethod=Integration: Trapezoidal  SampleTime=Ts  LimitOutput=on  UpperSaturationLimit=0.95  LowerSaturationLimit=-0.95  ICPrevOutput=DiscIntNeverNeededParam  ICPrevScaledInput=DiscIntNeverNeededParam
  Integral gain : Gain  Gain=Ki  SaturateOnIntegerOverflow=on  OutDataTypeStr=Inherit: Same as input  ParamDataTypeStr=Inherit: Same as input
  Proportional gain : Gain  Gain=Kp  SaturateOnIntegerOverflow=on  OutDataTypeStr=Inherit: Same as input  ParamDataTypeStr=Inherit: Same as input
  Sum1 : Sum  Inputs=+-  InputSameDT=on  SaturateOnIntegerOverflow=on  OutDataTypeStr=Inherit: Same as first input
  Sum2 : Sum  InputSameDT=on  SaturateOnIntegerOverflow=on  OutDataTypeStr=Inherit: Same as first input
  Ec : Outport  InitialOutput=0  VectorParamsAs1DForOutWhenUnconnected=off
  wires:
  Proportional gain/1 -> Sum2/1
  Integral gain/1 -> Discrete-Time Integrator/1
  Sum1/1 -> Integral gain/1, Proportional gain/1
  UBus/1 -> Sum1/1
  Uref/1 -> Sum1/2
  Discrete-Time Integrator/1 -> Sum2/2
  Sum2/1 -> Ctrl sat./1
  Ctrl sat./1 -> Ec/1

== system FuzzyHYPFWMLI/Fuel Cell 1/100Vdc Boost DC//DC Converter (average value)/Duty Cycles ==
  Ec : Inport
  Add : Sum  Inputs=+-
  Bus Creator2 : BusCreator  Inputs=2
  Constant : Constant
  Duty Cycle : Fcn  Expr=0.5*(u[1]+1)
  dc : Outport  VectorParamsAs1DForOutWhenUnconnected=off
  wires:
  Duty Cycle/1 -> Add/2, Bus Creator2/1  "IGBT I"
  Add/1 -> Bus Creator2/2  "IGBT 2"
  Constant/1 -> Add/1
  Ec/1 -> Duty Cycle/1
  Bus Creator2/1 -> dc/1
